simulink model "dyn_model"  (R2015a)
settings: Solver=ode45  StartTime=0.0  StopTime=tfin  FixedStep=Ts  RelTol=1e-3
values from neighbouring files (symbols this model uses):
  par = [1 5 1.5 4 20 0.5 1 0.5]    [main.m]
  x0 = zeros(size(Ad,1),1)    [LQI_control.m]    (also in main.m = [0 0 0 0]')
settings Model: CovSFcnEnable=off  Creator=dfamul  LastModifiedBy=Piero
settings DataIOCC: ExternalInput=[0 0]  InitialState=[]  LoadExternalInput=on  LoadInitialState=on  SignalLoggingSaveFormat=ModelDataLogs
settings OptimizationCC: InlineParams=on  BufferReuse=off  ExpressionDepthLimit=2147483647
settings DebuggingCC: UnderspecifiedInitializationDetection=Classic  MergeDetectMultiDrivingBlocksExec=none  FcnCallInpInsideContextMsg=EnableAllAsWarning  StateNameClashWarn=warning  InitInArrayFormatMsg=none
settings GRTTargetCC: CombineOutputUpdateFcns=off  GRTInterface=on
settings SimMechanicsCC: VisDuringSimulation=on

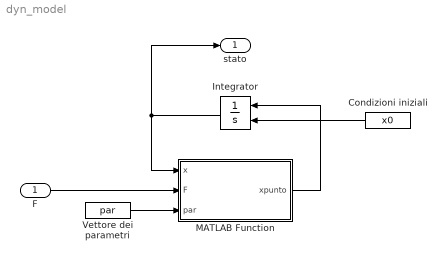
== system dyn_model ==
  "F " : Inport
  Condizioni iniziali : Constant  Value=x0
  Integrator : Integrator  InitialConditionSource=external  InitialCondition=x0
  MATLAB Function : MATLAB Function  TreatAsAtomicUnit=on
  Vettore dei parametri : Constant  Value=par
  stato : Outport
  wires:
  MATLAB Function/1(xpunto) -> Integrator/1
  "F "/1 -> MATLAB Function/2(F)
  Integrator/1 -> MATLAB Function/1(x), stato/1
  Vettore dei parametri/1 -> MATLAB Function/3(par)
  Condizioni iniziali/1 -> Integrator/2

== matlab function dyn_model/MATLAB Function ==
  data: x input; xpunto output; F input; par input
function xpunto = sys( x, F, par )

% Assegnazione paramentri
m1 = par(1);
k1 = par(2);
b1 = par(3);
m2 = par(4);
k2 = par(5);
b2 = par(6);
 L = par(7);
 R = par(8);

g = 9.81;

xpunto = zeros(4,1);
xpunto(1) = x(2);
xpunto(2) = -b1/(m1*L^2)*x(2) - k1/(m1*L^2)*(x(3)/R + x(1)) - g*cos(x(1))/L;
xpunto(3) = x(4);
xpunto(4) = -b2/m2*x(4) - k2/m2*x(3) - k1/(m2*R)*(x(3)/R + x(1)) - g + F/m2;

end
